simulink model "ct_sim"  (R2018b)
settings: Solver=VariableStepAuto  StartTime=0.0  StopTime=55  RelTol=1e-3
libraries: SignalEditorBlockLib x2
settings Model: Creator=EMiR  LastModifiedBy=EMiR
settings DataIOCC: OutputSaveName=out
settings OptimizationCC: DefaultUnderspecifiedDataType=single

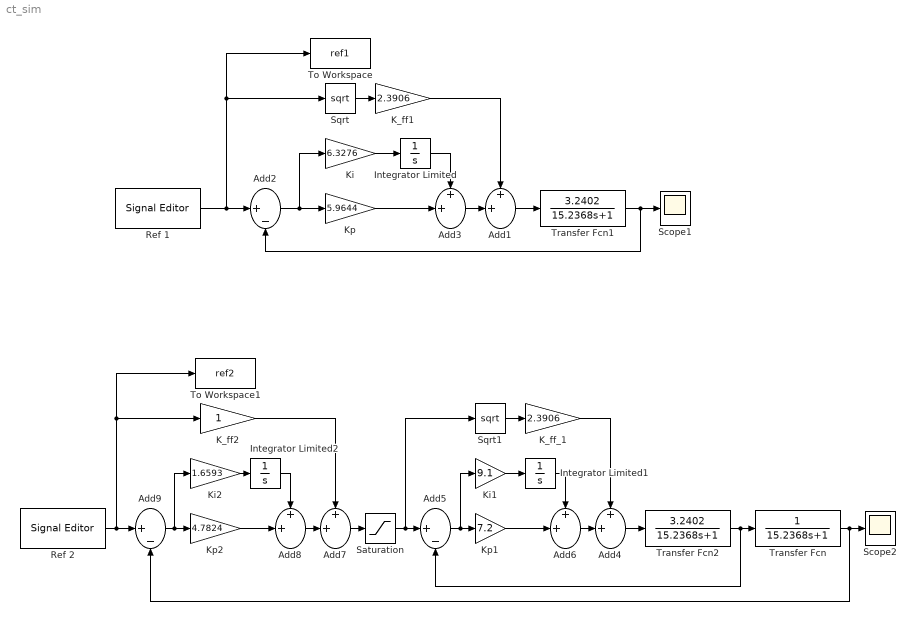
== system ct_sim ==
  Add{1,3..4,6..8} (6 alike) : Sum  Inputs=++|
  Add2 : Sum  Inputs=|+-
  Add5 : Sum  Inputs=|+-
  Add9 : Sum  Inputs=|+-
  Integrator Limited : Integrator  LimitOutput=on  UpperSaturationLimit=3.0  LowerSaturationLimit=-3.0
  Integrator Limited1 : Integrator  LimitOutput=on  UpperSaturationLimit=3.0  LowerSaturationLimit=-3.0
  Integrator Limited2 : Integrator  LimitOutput=on  UpperSaturationLimit=3.0  LowerSaturationLimit=-3.0
  K_ff1 : Gain  Gain=2.3906
  K_ff2 : Gain
  K_ff_1 : Gain  Gain=2.3906
  Ki : Gain  Gain=6.3276
  Ki1 : Gain  Gain=9.1
  Ki2 : Gain  Gain=1.6593
  Kp : Gain  Gain=5.9644
  Kp1 : Gain  Gain=7.2
  Kp2 : Gain  Gain=4.7824
  Ref 1 : SignalEditorBlockLib/Signal Editor  FileName=ref.mat  ActiveScenario=Scenario  ActiveSignal=Signal 1  IsBus=off  OutputBusObjectStr=Bus: BusObject  SampleTime=0  Interpolate=off  ZeroCross=off  OutputAfterFinalValue=Setting to zero  Unit=inherit
  Ref 2 : SignalEditorBlockLib/Signal Editor  FileName=ref2.mat  ActiveScenario=Scenario  ActiveSignal=Signal 1  IsBus=off  OutputBusObjectStr=Bus: BusObject  SampleTime=0  Interpolate=off  ZeroCross=off  OutputAfterFinalValue=Setting to zero  Unit=inherit
  Saturation : Saturate  UpperLimit=25.0  LowerLimit=-25.0
  Scope1 : Scope
  Scope2 : Scope
  Sqrt : Sqrt  SaturateOnIntegerOverflow=on
  Sqrt1 : Sqrt  SaturateOnIntegerOverflow=on
  To Workspace : ToWorkspace  VariableName=ref1  SampleTime=0.001
  To Workspace1 : ToWorkspace  VariableName=ref2  SampleTime=0.001
  Transfer Fcn : TransferFcn  Denominator=[15.2368 1]
  Transfer Fcn1 : TransferFcn  Numerator=[3.2402]  Denominator=[15.2368 1]
  Transfer Fcn2 : TransferFcn  Numerator=[3.2402]  Denominator=[15.2368 1]
  wires:
  Ref 1/1 -> Sqrt/1, To Workspace/1, Add2/1
  Sqrt/1 -> K_ff1/1
  K_ff1/1 -> Add1/1
  Add1/1 -> Transfer Fcn1/1
  Add3/1 -> Add1/2
  Kp/1 -> Add3/2
  Add2/1 -> Kp/1, Ki/1
  Ki/1 -> Integrator Limited/1
  Integrator Limited/1 -> Add3/1
  Kp1/1 -> Add6/2
  K_ff_1/1 -> Add4/1
  Add6/1 -> Add4/2
  Ki1/1 -> Integrator Limited1/1
  Integrator Limited1/1 -> Add6/1
  Add5/1 -> Kp1/1, Ki1/1
  Transfer Fcn2/1 -> Transfer Fcn/1, Add5/2
  Sqrt1/1 -> K_ff_1/1
  Add4/1 -> Transfer Fcn2/1
  Transfer Fcn/1 -> Scope2/1, Add9/2
  Kp2/1 -> Add8/2
  K_ff2/1 -> Add7/1
  Ki2/1 -> Integrator Limited2/1
  Integrator Limited2/1 -> Add8/1
  Add8/1 -> Add7/2
  Add9/1 -> Ki2/1, Kp2/1
  Ref 2/1 -> K_ff2/1, To Workspace1/1, Add9/1
  Add7/1 -> Saturation/1
  Saturation/1 -> Sqrt1/1, Add5/1
  Transfer Fcn1/1 -> Add2/2, Scope1/1
